simulink model "Environment_Gravity_TH"  (Simulink 7.4)
settings: Solver=ode45  StartTime=0.0  StopTime=10.0  RelTol=1e-3
libraries: AeroSim x2
settings Model: Creator=osborn_r  LastModifiedBy=osborn_r

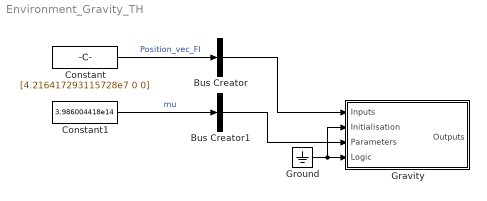
== system Environment_Gravity_TH ==
  Bus Creator : BusCreator  Inputs=1
  Bus Creator1 : BusCreator  Inputs=1
  Constant : Constant  Value=[4.216417293115728e7 0 0]  OutDataType=fixdt(1, 16)  OutScaling=2^0
  Constant1 : Constant  Value=3.986004418e14  OutDataType=fixdt(1, 16)  OutScaling=2^0
  Gravity : Subsystem
  Ground : Ground
  wires:
  Constant/1 -> Bus Creator/1  "Position_vec_FI"
  Constant1/1 -> Bus Creator1/1  "mu"
  Bus Creator/1 -> Gravity/1(Inputs)
  Bus Creator1/1 -> Gravity/3(Parameters)
  Ground/1 -> Gravity/4(Logic), Gravity/2(Initialisation)

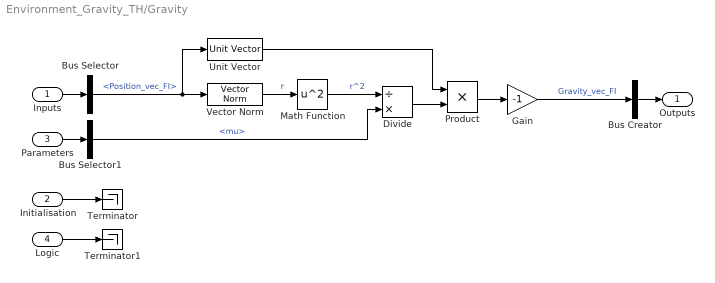
== system Environment_Gravity_TH/Gravity ==
  Inputs : Inport  OutDataType=fixdt(1, 16)  OutScaling=2^0
  Initialisation : Inport  Port=2  OutDataType=fixdt(1, 16)  OutScaling=2^0
  Parameters : Inport  Port=3  OutDataType=fixdt(1, 16)  OutScaling=2^0
  Logic : Inport  Port=4  OutDataType=fixdt(1, 16)  OutScaling=2^0
  Bus Creator : BusCreator  Inputs=1
  Bus Selector : BusSelector  OutputSignals=Position_vec_FI
  Bus Selector1 : BusSelector  OutputSignals=mu
  Divide : Product  Inputs=/*  OutDataType=fixdt(1, 16)  OutScaling=2^-10
  Gain : Gain  Gain=-1  ParameterDataType=fixdt(1, 16)  ParameterScaling=2^0  OutDataType=fixdt(1, 16)  OutScaling=2^0
  Math Function : Math  Operator=square  OutDataType=fixdt(1, 16)  OutScaling=2^0  SaturateOnIntegerOverflow=on
  Product : Product  OutDataType=fixdt(1, 16)  OutScaling=2^0  RndMeth=Zero
  Terminator : Terminator
  Terminator1 : Terminator
  Unit Vector : AeroSim/Mathematics/Unit Vector  SystemSampleTime=-1
  Vector Norm : AeroSim/Mathematics/Vector Norm  SystemSampleTime=-1
  Outputs : Outport  OutDataType=fixdt(1, 16)  OutScaling=2^0
  wires:
  Initialisation/1 -> Terminator/1
  Logic/1 -> Terminator1/1
  Inputs/1 -> Bus Selector/1
  Bus Selector/1 -> Vector Norm/1, Unit Vector/1  "<Position_vec_FI>"
  Vector Norm/1 -> Math Function/1  "r"
  Math Function/1 -> Divide/1  "r^2"
  Parameters/1 -> Bus Selector1/1
  Bus Selector1/1 -> Divide/2  "<mu>"
  Divide/1 -> Product/2
  Unit Vector/1 -> Product/1
  Product/1 -> Gain/1
  Bus Creator/1 -> Outputs/1
  Gain/1 -> Bus Creator/1  "Gravity_vec_FI"
